simulink model "system2"  (R2023b)
settings: Solver=FixedStepAuto  StartTime=0.0  StopTime=Tmdl  FixedStep=Tmdl/n_steps  RelTol=1e-3
undefined symbols (not defined in the file or in its folder): a1, a2, betta0, control_type, k, x1_initial, x2_initial
settings Model: Creator=deniskirbaba  LastModifiedBy=deniskirbaba

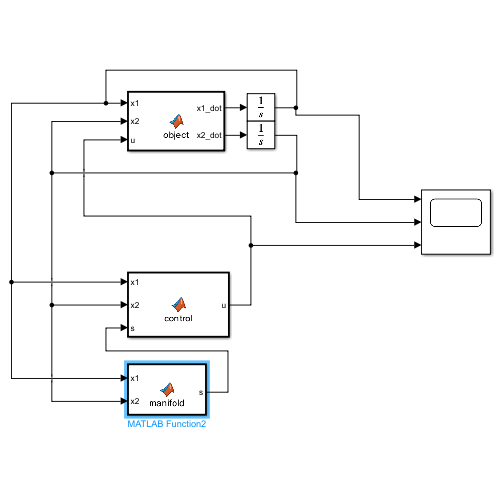
[thumbnail: Simulink's stored preview of the top-level diagram]
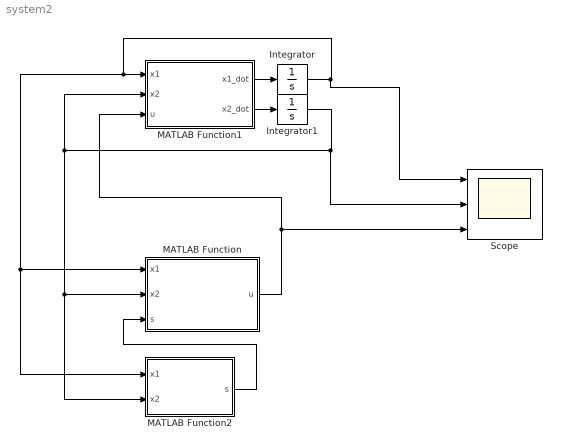
== system system2 ==
  Integrator : Integrator  InitialCondition=x1_initial
  Integrator1 : Integrator  InitialCondition=x2_initial
  MATLAB Function : MATLAB Function  TreatAsAtomicUnit=on
  MATLAB Function1 : MATLAB Function  TreatAsAtomicUnit=on
  MATLAB Function2 : MATLAB Function  TreatAsAtomicUnit=on
  Scope : Scope  NumInputPorts=3
  wires:
  MATLAB Function1/1(x1_dot) -> Integrator/1
  MATLAB Function1/2(x2_dot) -> Integrator1/1
  Integrator/1 -> Scope/1, MATLAB Function2/1(x1), MATLAB Function/1(x1), MATLAB Function1/1(x1)
  Integrator1/1 -> Scope/2, MATLAB Function1/2(x2), MATLAB Function2/2(x2), MATLAB Function/2(x2)
  MATLAB Function/1(u) -> Scope/3, MATLAB Function1/3(u)
  MATLAB Function2/1(s) -> MATLAB Function/3(s)

== matlab function system2/MATLAB Function1 ==
  data: x1 input; x2 input; u input; x1_dot output; x2_dot output; a1 parameter; a2 parameter
function [x1_dot, x2_dot] = object(x1,x2,u, a1, a2)

x1_dot = x2+a1*x1*sin(x1);
x2_dot = a2*x1*x2+3*u;

== matlab function system2/MATLAB Function ==
  data: x1 input; u output; x2 input; s input; betta0 parameter; control_type parameter; eps parameter; k parameter
function u = control(x1,x2,s, betta0,control_type, eps, k)

if control_type == 1
    u = -k*x2/3 - (abs(2*x1*x2+6*x1) + betta0)*(sign(s));
else
    sat_se = sign(s/eps);
    if abs(s/eps) <= 1
        sat_se = s/eps;
    end
    u = -k*x2/3 - (abs(2*x1*x2+6*x1) + betta0)*sat_se;
end

== matlab function system2/MATLAB Function2 ==
  data: x1 input; s output; x2 input; k parameter
function s = manifold(x1,x2, k)

s = x2+k*x1;
